simulink model "AGTF30SysSS"  (R2021b)
settings: Solver=FixedStepDiscrete  StartTime=0.0  StopTime=MWS.In.Max_IterSS  FixedStep=1  RelTol=1e-3  EnableMultiTasking=on
undefined symbols (not defined in the file): MWS
libraries: Lib_Cntrl_SetPoint_TMATS x2, Lib_Solve_SSNRSolverJC_TMATS x1
settings Model: Creator=jwchapm2  LastModifiedBy=prbalm
settings SolverCC: AlgebraicLoopSolver=TrustRegion
settings DataIOCC: LimitDataPoints=on  SaveFormat=Array  ReturnWorkspaceOutputs=off
settings OptimizationCC: LifeSpan=inf
settings DebuggingCC: SFUnexpectedBacktrackingDiag=warning  SFNoUnconditionalDefaultTransitionDiag=warning  SFExecutionAtInitializationDiag=none  SFMachineParentedDataDiag=warning  ArithmeticOperatorsInVariantConditions=warning
settings HardwareCC: ProdBitPerPointer=32  ProdBitPerSizeT=32  ProdBitPerPtrDiffT=32  ProdLargestAtomicFloat=None  ProdIntDivRoundTo=Undefined  ProdEndianess=Unspecified  ProdWordSize=32  ProdHWDeviceType=32-bit Generic
settings ModelReferenceCC: PropagateSignalLabelsOutOfModel=off
settings SFSimCC: SimUseLocalCustomCode=off  CustomCodeUndefinedFunction=UseInterfaceOnly
settings RTWCC: RTWUseLocalCustomCode=off
settings CodeAppCC: StateflowObjectComments=on
settings GRTTargetCC: TargetLangStandard=C89/C90 (ANSI)
settings ConfigComp: CovMetricSettings=dw  CovSaveCumulativeToWorkspaceVar=on  CovSaveSingleToWorkspaceVar=on  CovExternalEMLEnable=off

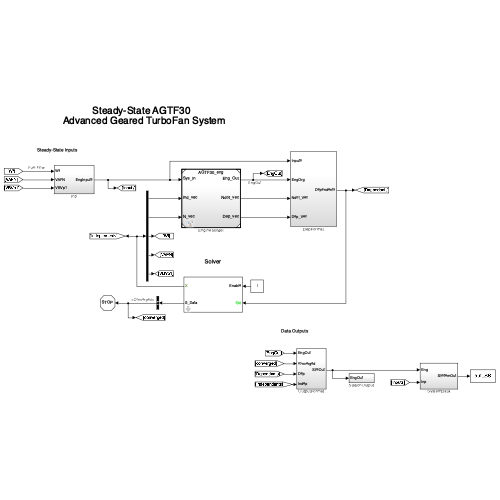
[thumbnail: Simulink's stored preview of the top-level diagram]
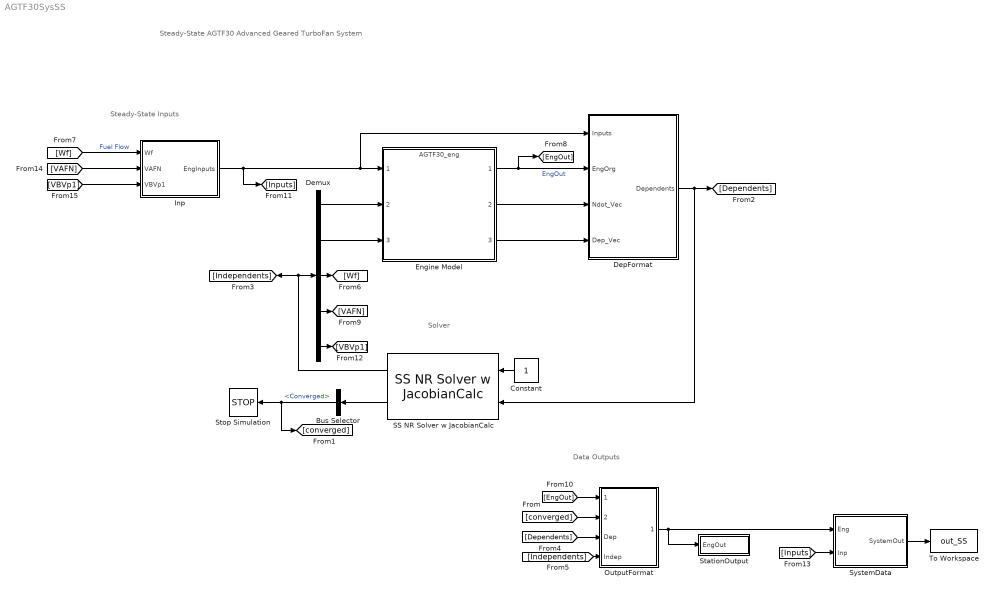
== system AGTF30SysSS ==
  note: Solver
  note: Steady-State Inputs
  note: Data Outputs
  note: Steady-State AGTF30
      | Advanced Geared TurboFan System
  Bus Selector : BusSelector  OutputSignals=Converged
  Constant : Constant
  Demux : Demux  Outputs=[7 2 1 1 1]
  DepFormat : Subsystem
  Engine Model : ModelReference  ModelNameDialog=AGTF30_eng.mdl  SimulationMode=Normal  ModelReferenceVersion=1.306
  Inp : Subsystem
  OutputFormat : Subsystem
  SS NR Solver w JacobianCalc : Lib_Solve_SSNRSolverJC_TMATS/SS NR Solver w JacobianCalc  SJac_Per_M=MWS.In.JPerSS  SNR_IC_M=[MWS.In.ICcom MWS.In.ICss]'  SNR_DX_M=1  SNR_Mx_M=1000000  SNR_Mn_M=0.000001  SJacobianAttempts_M=MWS.In.NRASS  Cond_Limits_M=MWS.In.Lim
  StationOutput : Subsystem
  Stop Simulation : Stop
  SystemData : Subsystem
  To Workspace : ToWorkspace  VariableName=out_SS  SaveFormat=Timeseries  SampleTime=-1
      settings: MaxDataPoints=1
  wires:
  Demux/2 -> Engine Model/3
  Demux/1 -> Engine Model/2
  Constant/1 -> SS NR Solver w JacobianCalc/1
  SS NR Solver w JacobianCalc/2 -> Bus Selector/1
  Bus Selector/1 -> Stop Simulation/1, [converged]  "<Converged>"
  Engine Model/1 -> [EngOut], DepFormat/2(EngOrg)  "EngOut"
  SS NR Solver w JacobianCalc/1 -> Demux/1, [Independents]
  Demux/3 -> [Wf]
  DepFormat/1(Dependents) -> SS NR Solver w JacobianCalc/2, [Dependents]
  Engine Model/2 -> DepFormat/3(Ndot_Vec)
  [converged] -> OutputFormat/2(converged)
  [Dependents] -> OutputFormat/3(Dep)
  [Independents] -> OutputFormat/4(Indep)
  [EngOut] -> OutputFormat/1(EngOut)
  Inp/1(EngInputs) -> [Inputs], DepFormat/1(Inputs), Engine Model/1
  [Wf] -> Inp/1(Wf)  "Fuel Flow"
  OutputFormat/1(SysOut) -> StationOutput/1(EngOut), SystemData/1(Eng)
  SystemData/1(SystemOut) -> To Workspace/1
  [Inputs] -> SystemData/2(Inp)
  Engine Model/3 -> DepFormat/4(Dep_Vec)
  [VAFN] -> Inp/2(VAFN)
  Demux/4 -> [VAFN]
  Demux/5 -> [VBVp1]
  [VBVp1] -> Inp/3(VBVp1)

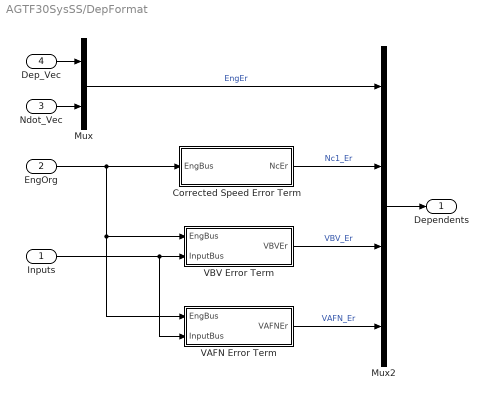
== system AGTF30SysSS/DepFormat ==
  Inputs : Inport
  EngOrg : Inport  Port=2
  Ndot_Vec : Inport  Port=3
  Dep_Vec : Inport  Port=4
  Corrected Speed Error Term : Subsystem
  Mux : Mux  Inputs=2
  Mux2 : Mux
  VAFN Error Term : Subsystem
  VBV Error Term : Subsystem
  Dependents : Outport
  wires:
  Ndot_Vec/1 -> Mux/2
  Mux/1 -> Mux2/1  "EngEr"
  Mux2/1 -> Dependents/1
  Dep_Vec/1 -> Mux/1
  Corrected Speed Error Term/1(NcEr) -> Mux2/2  "Nc1_Er"
  EngOrg/1 -> VAFN Error Term/1(EngBus), VBV Error Term/1(EngBus), Corrected Speed Error Term/1(EngBus)
  Inputs/1 -> VAFN Error Term/2(InputBus), VBV Error Term/2(InputBus)
  VBV Error Term/1(VBVEr) -> Mux2/3  "VBV_Er"
  VAFN Error Term/1(VAFNEr) -> Mux2/4  "VAFN_Er"

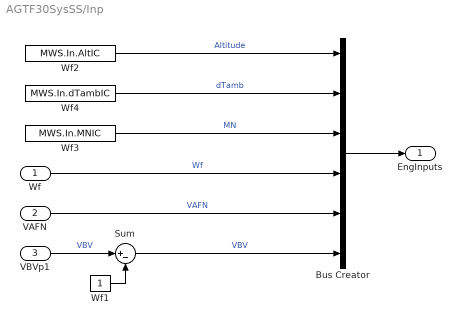
== system AGTF30SysSS/Inp ==
  Wf : Inport
  VAFN : Inport  Port=2
  VBVp1 : Inport  Port=3
  Bus Creator : BusCreator  Inputs=6
  Sum : Sum  Inputs=|+-
  Wf1 : Constant
  Wf2 : Constant  Value=MWS.In.AltIC
  Wf3 : Constant  Value=MWS.In.MNIC
  Wf4 : Constant  Value=MWS.In.dTambIC
  EngInputs : Outport
  wires:
  Wf2/1 -> Bus Creator/1  "Altitude"
  Wf3/1 -> Bus Creator/3  "MN"
  Bus Creator/1 -> EngInputs/1
  Sum/1 -> Bus Creator/6  "VBV"
  VAFN/1 -> Bus Creator/5  "VAFN"
  Wf4/1 -> Bus Creator/2  "dTamb"
  Wf/1 -> Bus Creator/4  "Wf"
  VBVp1/1 -> Sum/1  "VBV"
  Wf1/1 -> Sum/2

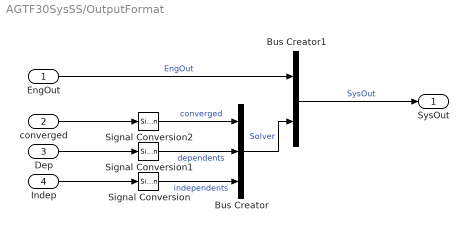
== system AGTF30SysSS/OutputFormat ==
  EngOut : Inport
  converged : Inport  Port=2
  Dep : Inport  Port=3
  Indep : Inport  Port=4
  Bus Creator : BusCreator  Inputs=3
  Bus Creator1 : BusCreator  Inputs=2
  Signal Conversion : SignalConversion  OverrideOpt=off
  Signal Conversion1 : SignalConversion  OverrideOpt=off
  Signal Conversion2 : SignalConversion  OverrideOpt=off
  SysOut : Outport
  wires:
  Signal Conversion1/1 -> Bus Creator/2  "dependents"
  Signal Conversion/1 -> Bus Creator/3  "independents"
  Signal Conversion2/1 -> Bus Creator/1  "converged"
  Bus Creator1/1 -> SysOut/1  "SysOut"
  Bus Creator/1 -> Bus Creator1/2  "Solver"
  Indep/1 -> Signal Conversion/1
  Dep/1 -> Signal Conversion1/1
  converged/1 -> Signal Conversion2/1
  EngOut/1 -> Bus Creator1/1  "EngOut"

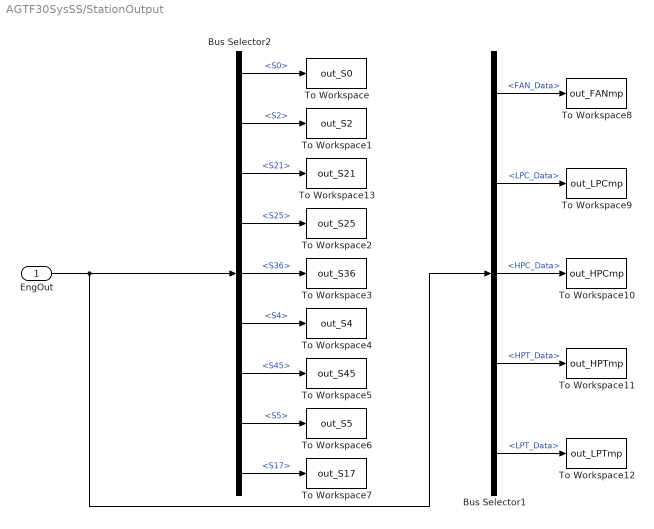
== system AGTF30SysSS/StationOutput ==
  EngOut : Inport
  Bus Selector1 : BusSelector  OutputSignals=EngOut.Data.FAN_Data,EngOut.Data.LPC_Data,EngOut.Data.HPC_Data,EngOut.Data.HPT_Data,EngOut.Data.LPT_Data
  Bus Selector2 : BusSelector  OutputSignals=EngOut.S0,EngOut.S2,EngOut.S21,EngOut.S25,EngOut.S36,EngOut.S4,EngOut.S45,EngOut.S5,EngOut.S17
  To Workspace : ToWorkspace  VariableName=out_S0  SaveFormat=Timeseries  SampleTime=-1
  To Workspace1 : ToWorkspace  VariableName=out_S2  SaveFormat=Timeseries  SampleTime=-1
  To Workspace10 : ToWorkspace  VariableName=out_HPCmp  SaveFormat=Timeseries  SampleTime=-1
  To Workspace11 : ToWorkspace  VariableName=out_HPTmp  SaveFormat=Timeseries  SampleTime=-1
  To Workspace12 : ToWorkspace  VariableName=out_LPTmp  SaveFormat=Timeseries  SampleTime=-1
  To Workspace13 : ToWorkspace  VariableName=out_S21  SaveFormat=Timeseries  SampleTime=-1
  To Workspace2 : ToWorkspace  VariableName=out_S25  SaveFormat=Timeseries  SampleTime=-1
  To Workspace3 : ToWorkspace  VariableName=out_S36  SaveFormat=Timeseries  SampleTime=-1
  To Workspace4 : ToWorkspace  VariableName=out_S4  SaveFormat=Timeseries  SampleTime=-1
  To Workspace5 : ToWorkspace  VariableName=out_S45  SaveFormat=Timeseries  SampleTime=-1
  To Workspace6 : ToWorkspace  VariableName=out_S5  SaveFormat=Timeseries  SampleTime=-1
  To Workspace7 : ToWorkspace  VariableName=out_S17  SaveFormat=Timeseries  SampleTime=-1
  To Workspace8 : ToWorkspace  VariableName=out_FANmp  SaveFormat=Timeseries  SampleTime=-1
  To Workspace9 : ToWorkspace  VariableName=out_LPCmp  SaveFormat=Timeseries  SampleTime=-1
  wires:
  Bus Selector1/5 -> To Workspace12/1  "<LPT_Data>"
  Bus Selector1/4 -> To Workspace11/1  "<HPT_Data>"
  Bus Selector1/3 -> To Workspace10/1  "<HPC_Data>"
  Bus Selector1/2 -> To Workspace9/1  "<LPC_Data>"
  Bus Selector1/1 -> To Workspace8/1  "<FAN_Data>"
  Bus Selector2/9 -> To Workspace7/1  "<S17>"
  Bus Selector2/8 -> To Workspace6/1  "<S5>"
  Bus Selector2/7 -> To Workspace5/1  "<S45>"
  Bus Selector2/6 -> To Workspace4/1  "<S4>"
  Bus Selector2/5 -> To Workspace3/1  "<S36>"
  Bus Selector2/4 -> To Workspace2/1  "<S25>"
  Bus Selector2/2 -> To Workspace1/1  "<S2>"
  EngOut/1 -> Bus Selector2/1, Bus Selector1/1
  Bus Selector2/1 -> To Workspace/1  "<S0>"
  Bus Selector2/3 -> To Workspace13/1  "<S21>"

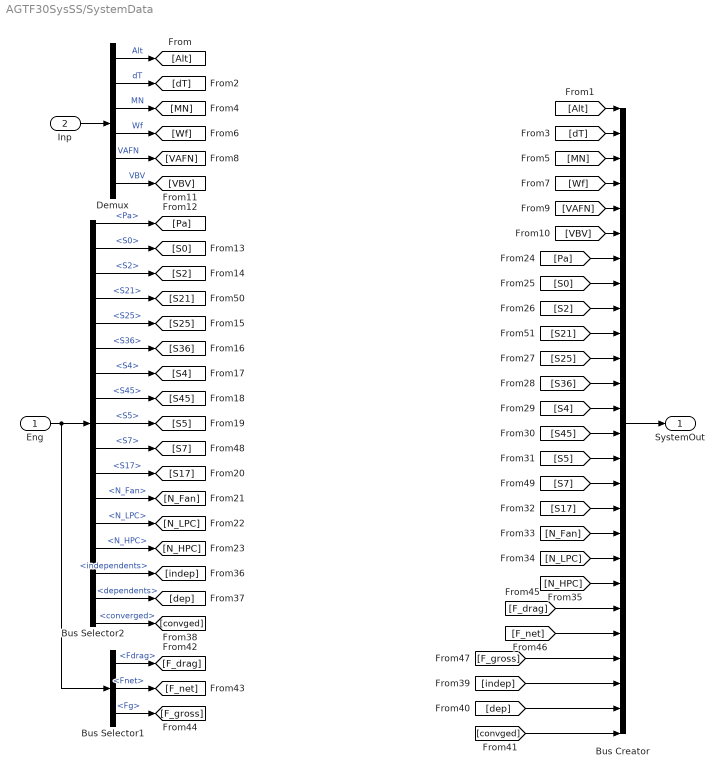
== system AGTF30SysSS/SystemData ==
  Eng : Inport
  Inp : Inport  Port=2
  Bus Creator : BusCreator  Inputs=26
  Bus Selector1 : BusSelector  OutputSignals=EngOut.Perf.Fdrag,EngOut.Perf.Fnet,EngOut.Perf.Fg
  Bus Selector2 : BusSelector  OutputSignals=EngOut.Amb.Pa,EngOut.S0,EngOut.S2,EngOut.S21,EngOut.S25,EngOut.S36,EngOut.S4,EngOut.S45,EngOut.S5,EngOut.S7,EngOut.S17,EngOut.Shaft.N_Fan,EngOut.Shaft.N_LPC,EngOut.Shaft.N_HPC,Solver.independents,Solver.dependents,Solver.converged
  Demux : Demux  Outputs=6
  SystemOut : Outport
  wires:
  Eng/1 -> Bus Selector1/1, Bus Selector2/1
  Bus Creator/1 -> SystemOut/1
  Inp/1 -> Demux/1
  [S2] -> Bus Creator/9
  [S0] -> Bus Creator/8
  [Pa] -> Bus Creator/7
  Demux/6 -> [VBV]  "VBV"
  Demux/5 -> [VAFN]  "VAFN"
  Demux/4 -> [Wf]  "Wf"
  Demux/3 -> [MN]  "MN"
  Demux/2 -> [dT]  "dT"
  Demux/1 -> [Alt]  "Alt"
  [Alt] -> Bus Creator/1
  [dT] -> Bus Creator/2
  [MN] -> Bus Creator/3
  [Wf] -> Bus Creator/4
  [VAFN] -> Bus Creator/5
  [VBV] -> Bus Creator/6
  Bus Selector2/1 -> [Pa]  "<Pa>"
  Bus Selector2/2 -> [S0]  "<S0>"
  Bus Selector2/3 -> [S2]  "<S2>"
  Bus Selector2/5 -> [S25]  "<S25>"
  Bus Selector2/6 -> [S36]  "<S36>"
  Bus Selector2/7 -> [S4]  "<S4>"
  Bus Selector2/8 -> [S45]  "<S45>"
  Bus Selector2/9 -> [S5]  "<S5>"
  Bus Selector2/11 -> [S17]  "<S17>"
  Bus Selector2/12 -> [N_Fan]  "<N_Fan>"
  Bus Selector2/13 -> [N_LPC]  "<N_LPC>"
  Bus Selector2/14 -> [N_HPC]  "<N_HPC>"
  Bus Selector2/15 -> [indep]  "<independents>"
  Bus Selector2/16 -> [dep]  "<dependents>"
  Bus Selector2/17 -> [convged]  "<converged>"
  Bus Selector1/1 -> [F_drag]  "<Fdrag>"
  Bus Selector1/2 -> [F_net]  "<Fnet>"
  Bus Selector1/3 -> [F_gross]  "<Fg>"
  Bus Selector2/10 -> [S7]  "<S7>"
  Bus Selector2/4 -> [S21]  "<S21>"
  [S21] -> Bus Creator/10
  [S4] -> Bus Creator/13
  [S45] -> Bus Creator/14
  [S17] -> Bus Creator/17
  [S5] -> Bus Creator/15
  [N_Fan] -> Bus Creator/18
  [S25] -> Bus Creator/11
  [S36] -> Bus Creator/12
  [S7] -> Bus Creator/16
  [N_LPC] -> Bus Creator/19
  [N_HPC] -> Bus Creator/20
  [F_drag] -> Bus Creator/21
  [F_net] -> Bus Creator/22
  [F_gross] -> Bus Creator/23
  [convged] -> Bus Creator/26
  [indep] -> Bus Creator/24
  [dep] -> Bus Creator/25

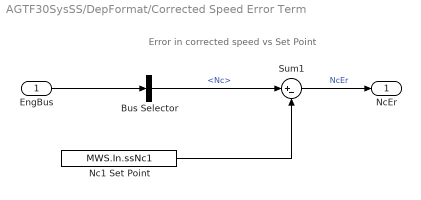
== system AGTF30SysSS/DepFormat/Corrected Speed Error Term ==
  note: Error in corrected speed vs Set Point
  EngBus : Inport
  Bus Selector : BusSelector  OutputSignals=Data.FAN_Data.Nc
  Nc1 Set Point : Constant  Value=MWS.In.ssNc1
  Sum1 : Sum  Inputs=|+-
  NcEr : Outport
  wires:
  Nc1 Set Point/1 -> Sum1/2
  Bus Selector/1 -> Sum1/1  "<Nc>"
  EngBus/1 -> Bus Selector/1
  Sum1/1 -> NcEr/1  "NcEr"

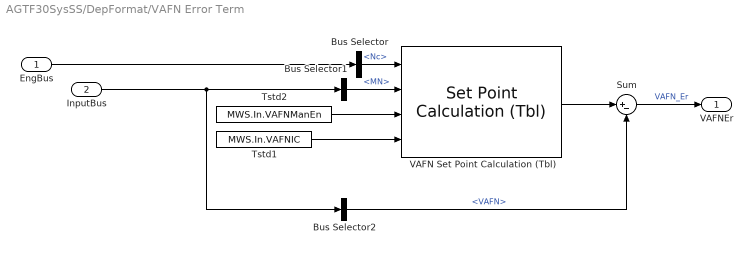
== system AGTF30SysSS/DepFormat/VAFN Error Term ==
  EngBus : Inport
  InputBus : Inport  Port=2
  Bus Selector : BusSelector  OutputSignals=Data.FAN_Data.Nc
  Bus Selector1 : BusSelector  OutputSignals=MN
  Bus Selector2 : BusSelector  OutputSignals=VAFN
  Sum : Sum  Inputs=|+-
  Tstd1 : Constant  Value=MWS.In.VAFNIC
  Tstd2 : Constant  Value=MWS.In.VAFNManEn
  VAFN Set Point Calculation (Tbl) : Lib_Cntrl_SetPoint_TMATS/Set Point Calculation (Tbl)  ERVec_M=MWS.Cntrl.VAFN_Nc1  DSVec_M=MWS.Cntrl.VAFN_MN  SPArray_M=MWS.Cntrl.VAFN_sch
  VAFNEr : Outport
  wires:
  Bus Selector2/1 -> Sum/2  "<VAFN>"
  InputBus/1 -> Bus Selector1/1, Bus Selector2/1
  Sum/1 -> VAFNEr/1  "VAFN_Er"
  Bus Selector/1 -> VAFN Set Point Calculation (Tbl)/1  "<Nc>"
  Tstd1/1 -> VAFN Set Point Calculation (Tbl)/4
  Tstd2/1 -> VAFN Set Point Calculation (Tbl)/3
  VAFN Set Point Calculation (Tbl)/1 -> Sum/1
  EngBus/1 -> Bus Selector/1
  Bus Selector1/1 -> VAFN Set Point Calculation (Tbl)/2  "<MN>"

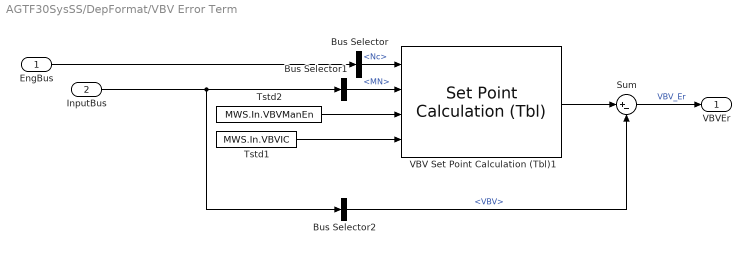
== system AGTF30SysSS/DepFormat/VBV Error Term ==
  EngBus : Inport
  InputBus : Inport  Port=2
  Bus Selector : BusSelector  OutputSignals=Data.FAN_Data.Nc
  Bus Selector1 : BusSelector  OutputSignals=MN
  Bus Selector2 : BusSelector  OutputSignals=VBV
  Sum : Sum  Inputs=|+-
  Tstd1 : Constant  Value=MWS.In.VBVIC
  Tstd2 : Constant  Value=MWS.In.VBVManEn
  VBV Set Point Calculation (Tbl)1 : Lib_Cntrl_SetPoint_TMATS/Set Point Calculation (Tbl)  ERVec_M=MWS.Cntrl.VBV_Nc1  DSVec_M=MWS.Cntrl.VBV_MN  SPArray_M=MWS.Cntrl.VBV_sch
  VBVEr : Outport
  wires:
  Bus Selector1/1 -> VBV Set Point Calculation (Tbl)1/2  "<MN>"
  EngBus/1 -> Bus Selector/1
  VBV Set Point Calculation (Tbl)1/1 -> Sum/1
  Tstd2/1 -> VBV Set Point Calculation (Tbl)1/3
  Tstd1/1 -> VBV Set Point Calculation (Tbl)1/4
  Bus Selector/1 -> VBV Set Point Calculation (Tbl)1/1  "<Nc>"
  Sum/1 -> VBVEr/1  "VBV_Er"
  InputBus/1 -> Bus Selector2/1, Bus Selector1/1
  Bus Selector2/1 -> Sum/2  "<VBV>"
